simulink model "obiekt_sterowanie"  (R2022b)
settings: Solver=VariableStepAuto  StartTime=0.0  StopTime=tmax  MaxStep=2  RelTol=1e-3
values from neighbouring files (symbols this model uses):
  Cpw = 1000    [obliczenia.m]    (also in obliczenia2.m)
  Cvg = Cmg*Rog*Vg    (= 501000)    [obliczenia.m]    (also in obliczenia2.m)
  Cvo1 = Cvg    (= 501000)    [obliczenia.m]    (also in obliczenia2.m)
  Cvo2 = Cvg    (= 501000)    [obliczenia.m]    (also in obliczenia2.m)
  Cvw = Cpw*Row*Vw*2    (= 288000)    [obliczenia.m]    (also in obliczenia2.m)
  dFmg1 = 0.05*Fmg10    (= 0.005)    [obliczenia.m]    (also in obliczenia2.m = 0)
  dFmg2 = 0    [obliczenia.m]    (also in obliczenia2.m)
  dQt1 = 0    [obliczenia.m]    (also in obliczenia2.m)
  dQt2 = 0    [obliczenia.m]    (also in obliczenia2.m)
  dTwew1 = 0    [obliczenia.m]    (also in obliczenia2.m)
  dTwz = 0    [obliczenia.m]    (also in obliczenia2.m)
  dTzew = 0    [obliczenia.m]    (also in obliczenia2.m)
  Fmg0 = FmgN*1.0    (= 0.1)    [obliczenia.m]    (also in obliczenia2.m)
  Fmw0 = FmwN    (= 0.2)    [obliczenia.m]    (also in obliczenia2.m)
  Kcg = QgN/(TgpN-TwewN)    (= 40)    [obliczenia.m]    (also in obliczenia2.m)
  Kco = 2*QgN/(TwpN-TozN)    (= 200)    [obliczenia.m]    (also in obliczenia2.m)
  Kcw = QgN/(TwewN-TzewN)    (= 50)    [obliczenia.m]    (also in obliczenia2.m)
  Ki = 0    [obliczenia2.m]
  Kp = Tczas1/(k1*Topu1)*6    (= 1.05226274907)    [obliczenia2.m]
  QtN = 0    [obliczenia.m]    (also in obliczenia2.m)
  SumT0 = (Tgp10*Fmg10 + Tgp20*Fmg20)/(Fmg10 + Fmg20)    (= 70)    [obliczenia.m]    (also in obliczenia2.m)
  T0 = 10    [obliczenia.m]    (also in obliczenia2.m)
  Tgp10 = ((Kcg + Kcw)*Twew10 - Kcw*Tzew0)/(Kcg)    (= 70)    [obliczenia.m]    (also in obliczenia2.m)
  Tgp20 = ((Kcg + Kcw)*Twew20 - Kcw*Tzew0)/(Kcg)    (= 70)    [obliczenia.m]    (also in obliczenia2.m)
  Tgz10 = TgzN + 0    (= 90)    [obliczenia.m]    (also in obliczenia2.m)
  Tgz20 = TgzN + 0    (= 90)    [obliczenia.m]    (also in obliczenia2.m)
  Ti = 3.33*TopuC/Kp    (= 11755.1763626)    [obliczenia2.m]
  Toz0 = TozN    (= 90)    [obliczenia.m]    (also in obliczenia2.m)
  tsok = 2000    [obliczenia.m]    (also in obliczenia2.m = 80000)
  Twew10 = (Cpw*Fmg10 *Kcg*Tgz10 + Kcw*(Kcg + Cpw*Fmg10)*Tzew0)/(Kcg*Kcw + Cpw*Fmg10*(Kcg + Kcw))    (= 20)    [obliczenia.m]    (also in obliczenia2.m)
  Twew20 = (Cpw*Fmg20 *Kcg*Tgz20 + Kcw*(Kcg + Cpw*Fmg20)*Tzew0)/(Kcg*Kcw + Cpw*Fmg20*(Kcg + Kcw))    (= 20)    [obliczenia.m]    (also in obliczenia2.m)
  TwewN = 20    [obliczenia.m]    (also in obliczenia2.m)
  Twp0 = TwpN    (= 110)    [obliczenia.m]    (also in obliczenia2.m)
  TwzN = 130    [obliczenia.m]    (also in obliczenia2.m)
  Tzew0 = TzewN + 0    (= -20)    [obliczenia.m]    (also in obliczenia2.m)
undefined symbols (not defined in the file or in its folder): tspadek
libraries: slpidlib x1
settings Model: Creator=asialalala  LastModifiedBy=asialalala
settings DataIOCC: ReturnWorkspaceOutputs=off

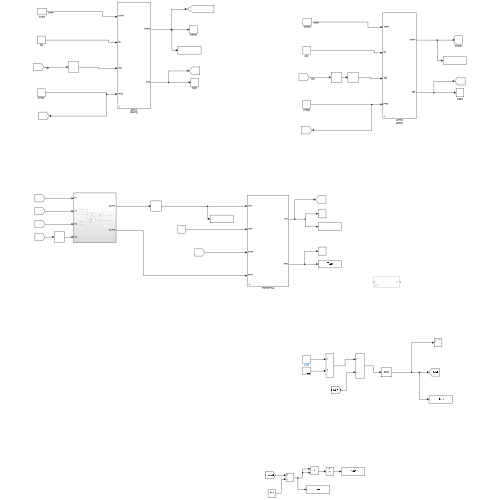
[thumbnail: Simulink's stored preview of the top-level diagram]
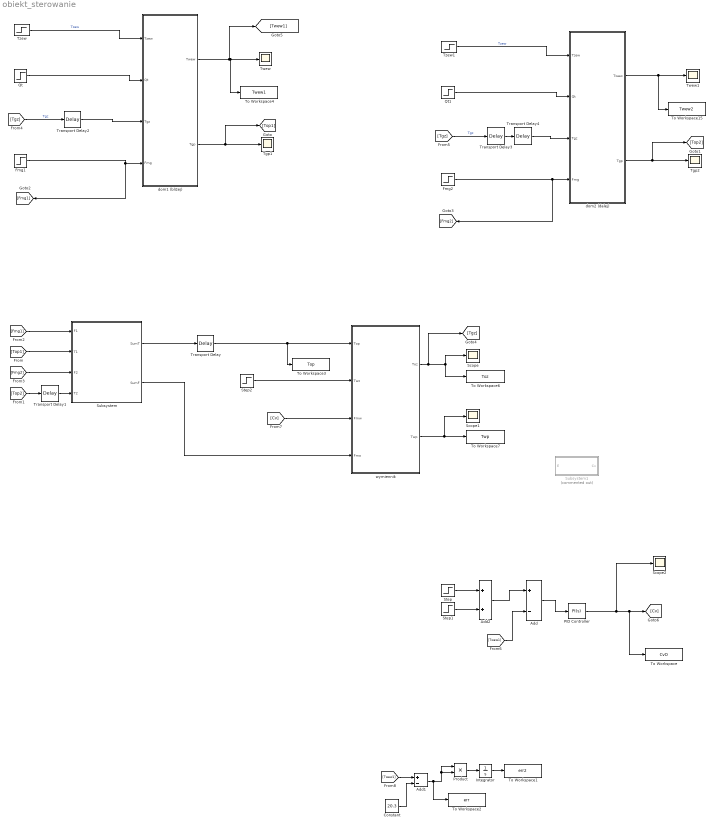
== system obiekt_sterowanie ==
  Add : Sum  Inputs=+-
  Add1 : Sum  Inputs=+-
  Add2 : Sum
  Constant : Constant  Value=20.3
  Fmg1 : Step  Time=tsok  Before=Fmg0  After=Fmg0 + dFmg1  SampleTime=0
  Fmg2 : Step  Time=tsok  Before=Fmg0  After=Fmg0 + dFmg2  SampleTime=0
  Integrator : Integrator
  PID Controller : slpidlib/PID Controller  Controller=PI  Form=Parallel  TimeDomain=Continuous-time  UseExternalTs=off  SampleTime=-1  IntegratorMethod=Forward Euler  FilterMethod=Forward Euler  ControllerParametersSource=internal  P=Kp  I=1/Ti  UseKiTs=off  D=0  N=100  UseFilter=on  TunerSelectOption=Transfer Function Based (PID Tuner App)  InitialConditionSource=internal  InitialConditionForIntegrator=Fmw0  InitialConditionForFilter=0  DifferentiatorICPrevScaledInput=0  ExternalReset=none  TrackingMode=off  Kt=1  LimitOutput=off  SatLimitsSource=internal  UpperSaturationLimit=inf  LowerSaturationLimit=-inf  LinearizeAsGain=on  AntiWindupMode=none  Kb=1  LimitIntegrator=off  UpperIntegratorSaturationLimit=inf  LowerIntegratorSaturationLimit=-inf  POutMin=[]  POutMax=[]  IOutMin=[]  IOutMax=[]  DOutMin=[]  DOutMax=[]  NOutMin=[]  NOutMax=[]  SumOutMin=[]  SumOutMax=[]  SaturationOutMin=[]  SaturationOutMax=[]  PParamMin=[]  PParamMax=[]  IParamMin=[]  IParamMax=[]  DParamMin=[]  DParamMax=[]  NParamMin=[]  NParamMax=[]  KbParamMin=[]  KbParamMax=[]  KtParamMin=[]  KtParamMax=[]  KbOutMin=[]  KbOutMax=[]  KtOutMin=[]  KtOutMax=[]  IntegratorOutMin=[]  IntegratorOutMax=[]  FilterOutMin=[]  FilterOutMax=[]  SumI1OutMin=[]  SumI1OutMax=[]  SumI2OutMin=[]  SumI2OutMax=[]  SumI3OutMin=[]  SumI3OutMax=[]  SumI4OutMin=[]  SumI4OutMax=[]  SumDOutMin=[]  SumDOutMax=[]  DifferentiatorOutMin=[]  DifferentiatorOutMax=[]  FilterDiffOutCoefMin=[]  FilterDiffOutCoefMax=[]  ReciprocalOutMin=[]  ReciprocalOutMax=[]  SumDenOutMin=[]  SumDenOutMax=[]  SumNumOutMin=[]  SumNumOutMax=[]  DivideOutMin=[]  DivideOutMax=[]  UdiffTsProdOutMin=[]  UdiffTsProdOutMax=[]  NTsProdOutMin=[]  NTsProdOutMax=[]  UintegralTsProdOutMin=[]  UintegralTsProdOutMax=[]  UngainTsProdOutMin=[]  UngainTsProdOutMax=[]  ClampingZeroOutDataTypeStr=Inherit: Inherit via back propagation  ClampingZeroOutMin=[]  ClampingZeroOutMax=[]  FilterDenConstantOutDataTypeStr=Inherit: Inherit via back propagation  FilterDenConstantOutMin=[]  FilterDenConstantOutMax=[]  PCopyOutDataTypeStr=Inherit: Inherit via back propagation  PCopyOutMin=[]  PCopyOutMax=[]  NCopyOutDataTypeStr=Inherit: Inherit via back propagation  NCopyOutMin=[]  NCopyOutMax=[]  IntegratorContinuousStateAttributes=''  IntegratorStateMustResolveToSignalObject=off  IntegratorRTWStateStorageClass=Auto  FilterContinuousStateAttributes=''  FilterStateMustResolveToSignalObject=off  FilterRTWStateStorageClass=Auto  ParallelPVariant=InternalParameters  IdealPVariant=Disabled  IVariant=InternalParameters  DVariant=Disabled  IntegratorVariant=Continuous  SatVariant=Disabled  AWVariant=Passthrough  PCopyVariant=Disabled  TRVariant=Disabled  FdbkBlocksVariant=Forward  IdealPFdbkVariant=Disabled  SatFdbkVariant=Disabled  DerivativeFilterVariant=Disabled  NVariant=Disabled  NCopyVariant=Disabled_SignalSpec  FilterICVariant=Disabled  IntegratorICVariant=InternalICs  ExternalResetVariant=Disabled  TRSumVariant=Passthrough  SumFdbkVariant=Disabled  SumVariant=Sum_PI  TsampFilterVariant=InternalTs  TsampNgainVariant=Passthrough  TsampIntegralVariant=Passthrough  ExternalSaturationOutDataTypeStr=Inherit: Same as second input
  Product : Product
  Qt : Step  Time=tsok  Before=QtN  After=QtN + dQt1  SampleTime=0
  Qt1 : Step  Time=tsok  Before=QtN  After=QtN + dQt2  SampleTime=0
  Scope : Scope
  Scope1 : Scope
  Scope2 : Scope
  Step : Step  Time=tsok  Before=TwewN  After=TwewN + dTwew1  SampleTime=0
  Step1 : Step  Time=tspadek  After=-dTwew1  SampleTime=0
  Step2 : Step  Time=tsok  Before=TwzN  After=TwzN + dTwz  SampleTime=0
  Subsystem : Subsystem
  Subsystem1 : Subsystem  Commented=on  mask{Kp=Kp, Ti=Ti, Cv0=Fmw0, Ki=Ki}
  Tgp1 : Scope
  Tgp2 : Scope
  To Workspace : ToWorkspace  VariableName=CvO  SampleTime=-1
  To Workspace1 : ToWorkspace  VariableName=err2  SampleTime=-1
      settings: Save2DSignal=2-D array (concatenate along first dimension)
  To Workspace15 : ToWorkspace  VariableName=Twew2  SampleTime=-1
  To Workspace2 : ToWorkspace  VariableName=err  SampleTime=-1
      settings: Save2DSignal=2-D array (concatenate along first dimension)
  To Workspace3 : ToWorkspace  VariableName=Top  SaveFormat=Timeseries  SampleTime=-1
  To Workspace4 : ToWorkspace  VariableName=Twew1  SampleTime=-1
  To Workspace6 : ToWorkspace  VariableName=Toz  SampleTime=-1
  To Workspace7 : ToWorkspace  VariableName=Twp  SampleTime=-1
  Transport Delay : TransportDelay  DelayTime=T0  InitialOutput=SumT0
  Transport Delay1 : TransportDelay  DelayTime=T0  InitialOutput=Tgp20
  Transport Delay2 : TransportDelay  DelayTime=T0  InitialOutput=Tgz10
  Transport Delay3 : TransportDelay  DelayTime=T0  InitialOutput=Tgz20
  Transport Delay4 : TransportDelay  DelayTime=T0  InitialOutput=Tgz20
  Twew : Scope
  Twew1 : Scope
  Tzew : Step  Time=tsok  Before=Tzew0  After=Tzew0 + dTzew  SampleTime=0
  Tzew1 : Step  Time=tsok  Before=Tzew0  After=Tzew0 + dTzew  SampleTime=0
  dom1 (bliżej) : Subsystem  mask{Kcw=Kcw, Kcg=Kcg, Cvw=Cvw, Cvg=Cvg, Cpw=Cpw}
  dom2 (dalej) : Subsystem  mask{Kcw=Kcw, Kcg=Kcg, Cvw=Cvw, Cvg=Cvg, Cpw=Cpw}
  wymiennik : Subsystem  mask{Cvo1=Cvo1, Cvo2=Cvo2, Kco=Kco}
  wires:
  Tzew/1 -> dom1 (bliżej)/1(Tzew)  "Tzew"
  Qt/1 -> dom1 (bliżej)/2(Qt)
  dom1 (bliżej)/1(Twew) -> [Twew1], Twew/1, To Workspace4/1
  dom1 (bliżej)/2(Tgp) -> [Top1], Tgp1/1
  wymiennik/1(Toz) -> [Tgz], Scope/1, To Workspace6/1
  wymiennik/2(Twp) -> Scope1/1, To Workspace7/1
  Step2/1 -> wymiennik/2(Twz)
  Subsystem/1(SumT) -> Transport Delay/1
  Tzew1/1 -> dom2 (dalej)/1(Tzew)  "Tzew"
  dom2 (dalej)/2(Tgp) -> [Top2], Tgp2/1
  Qt1/1 -> dom2 (dalej)/2(Qt)
  dom2 (dalej)/1(Twew) -> Twew1/1, To Workspace15/1
  [Top1] -> Subsystem/2(T1)
  [Fmg1] -> Subsystem/1(F1)
  Subsystem/2(SumF) -> wymiennik/4(Fmo)
  [Fmg2] -> Subsystem/3(F2)
  Fmg1/1 -> [Fmg1], dom1 (bliżej)/4(Fmg)
  Fmg2/1 -> [Fmg2], dom2 (dalej)/4(Fmg)
  [Top2] -> Transport Delay1/1
  Transport Delay3/1 -> Transport Delay4/1
  [Tgz] -> Transport Delay2/1  "Tgz"
  Transport Delay2/1 -> dom1 (bliżej)/3(Tgz)
  Transport Delay4/1 -> dom2 (dalej)/3(Tgz)
  [Tgz] -> Transport Delay3/1  "Tgz"
  Transport Delay/1 -> To Workspace3/1, wymiennik/1(Top)
  Transport Delay1/1 -> Subsystem/4(T2)
  [Cv] -> wymiennik/3(Fmw)
  [Twew1] -> Add/2
  Integrator/1 -> To Workspace1/1
  [Twew1] -> Add1/1
  Add1/1 -> To Workspace2/1, Product/2, Product/1
  Product/1 -> Integrator/1
  Constant/1 -> Add1/2
  Add/1 -> PID Controller/1
  PID Controller/1 -> Scope2/1, To Workspace/1, [Cv]
  Step/1 -> Add2/1
  Add2/1 -> Add/1
  Step1/1 -> Add2/2

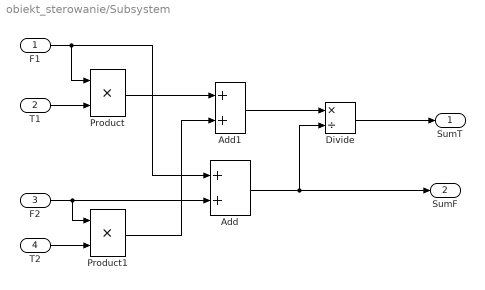
== system obiekt_sterowanie/Subsystem ==
  F1 : Inport
  T1 : Inport  Port=2
  F2 : Inport  Port=3
  T2 : Inport  Port=4
  Add : Sum
  Add1 : Sum
  Divide : Product  Inputs=*/
  Product : Product
  Product1 : Product
  SumT : Outport
  SumF : Outport  Port=2
  wires:
  Add/1 -> Divide/2, SumF/1
  F2/1 -> Add/2, Product1/1
  F1/1 -> Product/1, Add/1
  T1/1 -> Product/2
  T2/1 -> Product1/2
  Product1/1 -> Add1/2
  Product/1 -> Add1/1
  Add1/1 -> Divide/1
  Divide/1 -> SumT/1

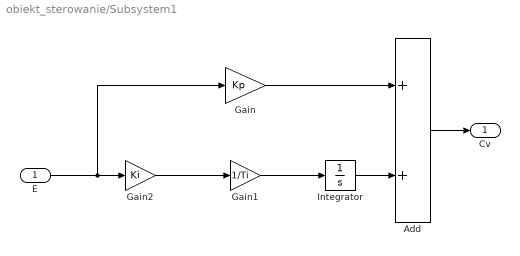
== system obiekt_sterowanie/Subsystem1 ==
  E : Inport
  Add : Sum
  Gain : Gain  Gain=Kp
  Gain1 : Gain  Gain=1/Ti
  Gain2 : Gain  Gain=Ki
  Integrator : Integrator  InitialCondition=Cv0
  Cv : Outport
  wires:
  Gain2/1 -> Gain1/1
  Gain1/1 -> Integrator/1
  E/1 -> Gain/1, Gain2/1
  Integrator/1 -> Add/2
  Add/1 -> Cv/1
  Gain/1 -> Add/1

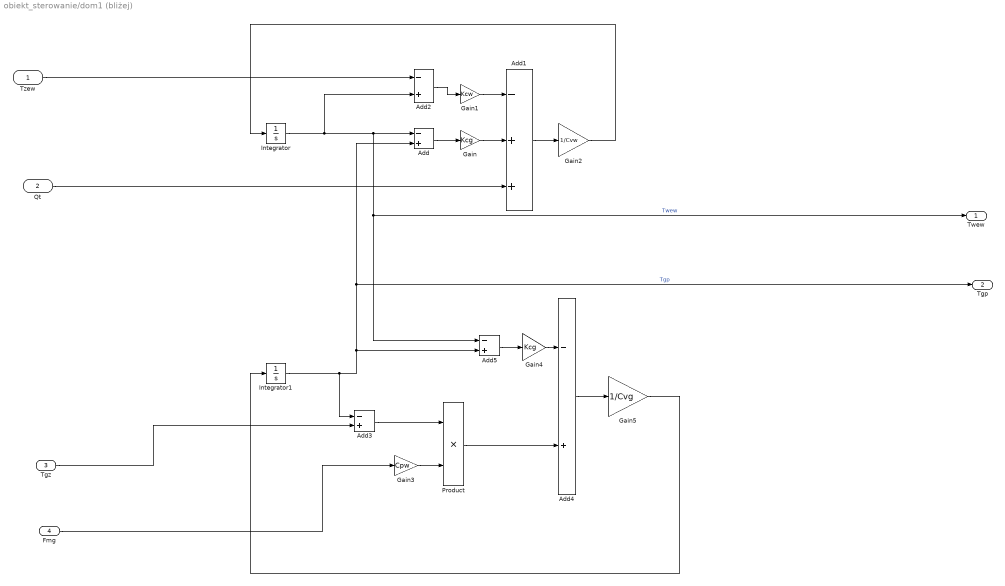
== system obiekt_sterowanie/dom1 (bliżej) ==
  Tzew : Inport
  Qt : Inport  Port=2
  Tgz : Inport  Port=3
  Fmg : Inport  Port=4
  Add{,2..5} (5 alike) : Sum  Inputs=-+
  Add1 : Sum  Inputs=-++
  Gain : Gain  Gain=Kcg
  Gain1 : Gain  Gain=Kcw
  Gain2 : Gain  Gain=1/Cvw
  Gain3 : Gain  Gain=Cpw
  Gain4 : Gain  Gain=Kcg
  Gain5 : Gain  Gain=1/Cvg
  Integrator : Integrator  InitialCondition=Twew10
  Integrator1 : Integrator  InitialCondition=Tgp10
  Product : Product
  Twew : Outport
  Tgp : Outport  Port=2
  wires:
  Fmg/1 -> Gain3/1
  Add/1 -> Gain/1
  Gain3/1 -> Product/2
  Qt/1 -> Add1/3
  Product/1 -> Add4/2
  Gain2/1 -> Integrator/1
  Add2/1 -> Gain1/1
  Add5/1 -> Gain4/1
  Integrator1/1 -> Add3/1, Add5/2, Tgp/1, Add/2  "Tgp"
  Integrator/1 -> Add2/2, Twew/1, Add5/1, Add/1  "Twew"
  Gain/1 -> Add1/2
  Gain4/1 -> Add4/1
  Gain1/1 -> Add1/1
  Tzew/1 -> Add2/1
  Add3/1 -> Product/1
  Gain5/1 -> Integrator1/1
  Add4/1 -> Gain5/1
  Add1/1 -> Gain2/1
  Tgz/1 -> Add3/2

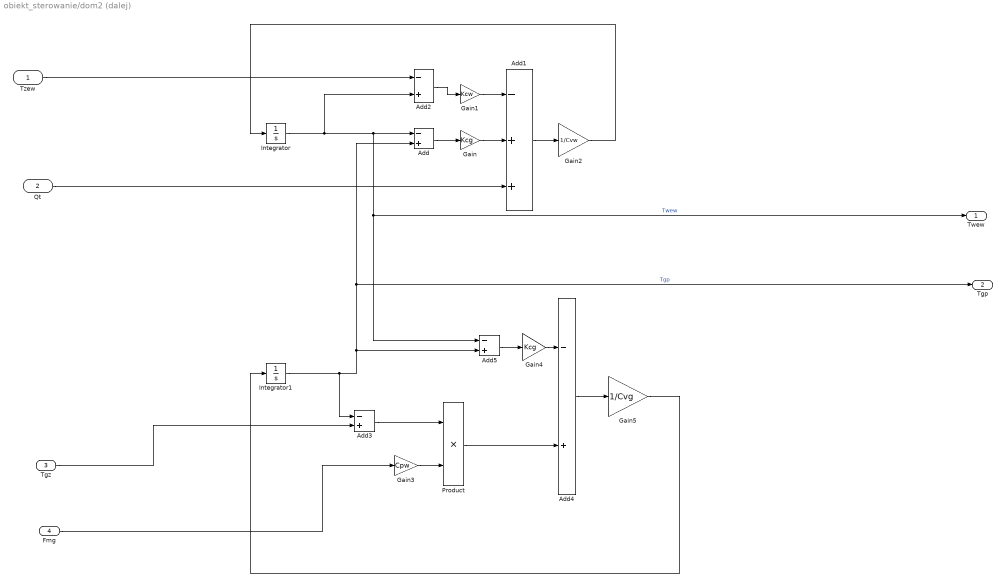
== system obiekt_sterowanie/dom2 (dalej) ==
  Tzew : Inport
  Qt : Inport  Port=2
  Tgz : Inport  Port=3
  Fmg : Inport  Port=4
  Add{,2..5} (5 alike) : Sum  Inputs=-+
  Add1 : Sum  Inputs=-++
  Gain : Gain  Gain=Kcg
  Gain1 : Gain  Gain=Kcw
  Gain2 : Gain  Gain=1/Cvw
  Gain3 : Gain  Gain=Cpw
  Gain4 : Gain  Gain=Kcg
  Gain5 : Gain  Gain=1/Cvg
  Integrator : Integrator  InitialCondition=Twew20
  Integrator1 : Integrator  InitialCondition=Tgp20
  Product : Product
  Twew : Outport
  Tgp : Outport  Port=2
  wires:
  Fmg/1 -> Gain3/1
  Add/1 -> Gain/1
  Gain3/1 -> Product/2
  Qt/1 -> Add1/3
  Product/1 -> Add4/2
  Gain2/1 -> Integrator/1
  Add2/1 -> Gain1/1
  Add5/1 -> Gain4/1
  Integrator1/1 -> Add3/1, Add5/2, Tgp/1, Add/2  "Tgp"
  Integrator/1 -> Add2/2, Twew/1, Add5/1, Add/1  "Twew"
  Gain/1 -> Add1/2
  Gain4/1 -> Add4/1
  Gain1/1 -> Add1/1
  Tzew/1 -> Add2/1
  Add3/1 -> Product/1
  Gain5/1 -> Integrator1/1
  Add4/1 -> Gain5/1
  Add1/1 -> Gain2/1
  Tgz/1 -> Add3/2

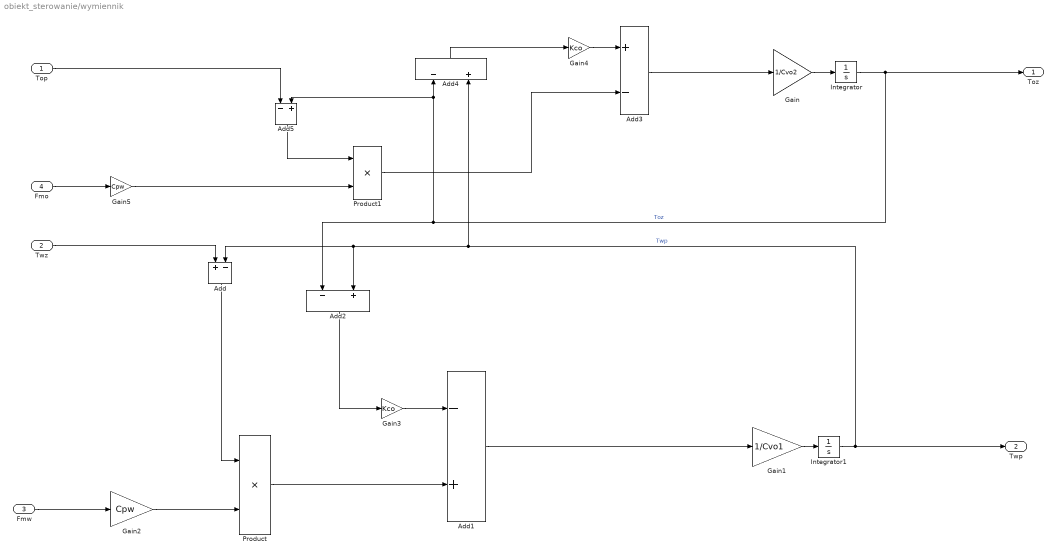
== system obiekt_sterowanie/wymiennik ==
  Top : Inport
  Twz : Inport  Port=2
  Fmw : Inport  Port=3
  Fmo : Inport  Port=4
  Add : Sum  Inputs=+-
  Add{1..2,4..5} (4 alike) : Sum  Inputs=-+
  Add3 : Sum  Inputs=+-
  Gain : Gain  Gain=1/Cvo2
  Gain1 : Gain  Gain=1/Cvo1
  Gain2 : Gain  Gain=Cpw
  Gain3 : Gain  Gain=Kco
  Gain4 : Gain  Gain=Kco
  Gain5 : Gain  Gain=Cpw
  Integrator : Integrator  InitialCondition=Toz0
  Integrator1 : Integrator  InitialCondition=Twp0
  Product : Product
  Product1 : Product
  Toz : Outport
  Twp : Outport  Port=2
  wires:
  Integrator/1 -> Add2/1, Add5/2, Add4/1, Toz/1  "Toz"
  Integrator1/1 -> Twp/1, Add/2, Add2/2, Add4/2  "Twp"
  Gain/1 -> Integrator/1
  Gain1/1 -> Integrator1/1
  Fmw/1 -> Gain2/1
  Twz/1 -> Add/1
  Gain2/1 -> Product/2
  Add/1 -> Product/1
  Product/1 -> Add1/2
  Gain3/1 -> Add1/1
  Add2/1 -> Gain3/1
  Add1/1 -> Gain1/1
  Add3/1 -> Gain/1
  Gain4/1 -> Add3/1
  Add4/1 -> Gain4/1
  Fmo/1 -> Gain5/1
  Gain5/1 -> Product1/2
  Add5/1 -> Product1/1
  Product1/1 -> Add3/2
  Top/1 -> Add5/1
